simulink model "reto12"  (R2024a)
settings: Solver=VariableStepAuto  StartTime=0.0  StopTime=10.0  RelTol=1e-3
settings Model: Creator=Usuario  LastModifiedBy=Usuario

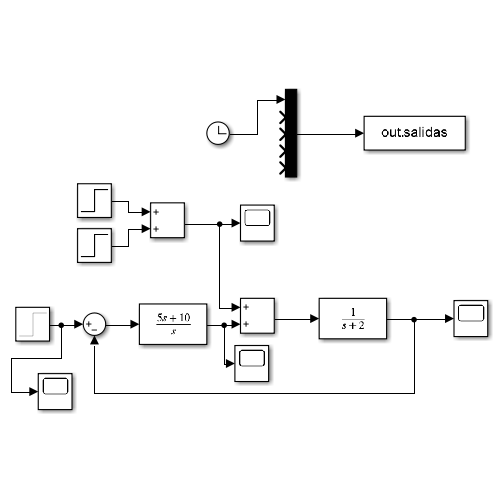
[thumbnail: Simulink's stored preview of the top-level diagram]
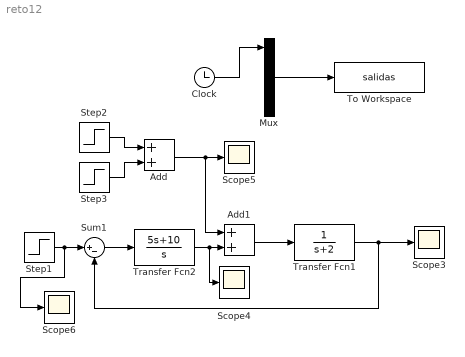
== system reto12 ==
  Add : Sum
  Add1 : Sum
  Clock : Clock
  Mux : Mux  Inputs=5
  Scope{3..6} (4 alike) : Scope
  Step1 : Step  Time=0  SampleTime=0
  Step2 : Step  Time=0  After=3  SampleTime=0
  Step3 : Step  Time=3  After=5  SampleTime=0
  Sum1 : Sum  Inputs=|+-
  To Workspace : ToWorkspace  VariableName=salidas  SampleTime=-1
  Transfer Fcn1 : TransferFcn  Denominator=[1 2]
  Transfer Fcn2 : TransferFcn  Numerator=[5 10]  Denominator=[1 0]
  wires:
  Add/1 -> Scope5/1, Add1/1
  Transfer Fcn2/1 -> Scope4/1, Add1/2
  Step3/1 -> Add/2
  Sum1/1 -> Transfer Fcn2/1
  Step2/1 -> Add/1
  Transfer Fcn1/1 -> Sum1/2, Scope3/1
  Mux/1 -> To Workspace/1
  Clock/1 -> Mux/1
  Add1/1 -> Transfer Fcn1/1
  Step1/1 -> Scope6/1, Sum1/1
